simulink library "LM_LIB"  (R2019b)
settings: Solver=VariableStepAuto  StartTime=0.0  StopTime=10.0  RelTol=1e-3
undefined symbols (not defined in the file): P_LM_FusBLParFiltP, P_LM_FusParC0Index, P_LM_FusParC1Index, P_LM_FusParC2Index, P_LM_FusParC3Index, P_LM_OTLBufTPMinPntNum, P_LM_OTLBufTPSPosMinDis, P_LM_OTLRearMaxDis, P_LM_OTLTPNum
libraries: simulink x84, $bdroot x3
(part 4 of 5)

== system LM_LIB/LM_OTL_Buf2InfoUpdate/LM_OTL_BufLe1StoreInfoCalc/LM_OTL_ObjSICCurLeObj1InBufLe1 ==
  LM_OTLCurLeLaObj1RcdFlg : Inport
  LM_OTLCurLeLaObj1ID : Inport  Port=2
  LM_OTLCurLeLaObj1Dx : Inport  Port=3
  LM_OTLCurLeLaObj1Dy : Inport  Port=4
  LM_OTLBufL1PNumK1 : Inport  Port=5
  LM_OTLBufL1SPPosK1 : Inport  Port=6
  LM_OTLBufL1EPPosK1 : Inport  Port=7
  LM_OTLBufDxVectK1Adju : Inport  Port=8
  Action Port : ActionPort
  LM_OTL_BufL1DxInfo : Subsystem
  LM_OTL_BufL1DyInfo : Subsystem
  LM_OTL_BufL1EPInfo : Subsystem
  LM_OTL_BufL1IDInfo : Subsystem
  LM_OTL_BufL1PNumAndSPInfo : $bdroot/LM_OTL_Buf1InfoUpdate/LM_OTL_BufLe1StoreInfoCalc/LM_OTL_ObjSICCurLeObj1InBufLe1/LM_OTL_BufL1PNumAndSPInfo  SystemSampleTime=-1  Latency=0  AutoFrameSizeCalculation=off
  LM_OTL_BufL1UpdateFlg : Subsystem
  LM_OTLBufL1UpdateFlg : Outport
  LM_OTLBufL1ObjID : Outport  Port=2
  LM_OTLBufL1Objdx : Outport  Port=3
  LM_OTLBufL1Objdy : Outport  Port=4
  LM_OTLBufL1ObjTPNum : Outport  Port=5
  LM_OTLBufL1ObjTPSP : Outport  Port=6
  LM_OTLBufL1ObjTPEP : Outport  Port=7
  wires:
  LM_OTL_BufL1EPInfo/1(LM_OTLBufL1EPPos) -> LM_OTLBufL1ObjTPEP/1, [LM_OTLBufL1EPPos]
  [LM_OTLBufL1EPPos] -> LM_OTL_BufL1PNumAndSPInfo/4
  LM_OTL_BufL1IDInfo/1(LM_OTLBufL1ObjID) -> LM_OTLBufL1ObjID/1
  LM_OTL_BufL1DxInfo/1(LM_OTLBufL1Objdx) -> LM_OTLBufL1Objdx/1
  LM_OTL_BufL1DyInfo/1(LM_OTLBufL1ObjDy) -> LM_OTLBufL1Objdy/1
  LM_OTL_BufL1PNumAndSPInfo/1 -> LM_OTLBufL1ObjTPNum/1
  LM_OTL_BufL1PNumAndSPInfo/2 -> LM_OTLBufL1ObjTPSP/1
  LM_OTL_BufL1UpdateFlg/1(LM_OTLBufL1UpdateFlg) -> LM_OTLBufL1UpdateFlg/1
  LM_OTLCurLeLaObj1RcdFlg/1 -> LM_OTL_BufL1EPInfo/1(LM_OTLCurLeLaObj1RcdFlg), LM_OTL_BufL1PNumAndSPInfo/2, LM_OTL_BufL1DyInfo/2(LM_OTLCurLeLaObj1RcdFlg), LM_OTL_BufL1DxInfo/2(LM_OTLCurLeLaObj1RcdFlg), LM_OTL_BufL1UpdateFlg/1(LM_OTLCurLeLaObj1RcdFlg)
  LM_OTLCurLeLaObj1ID/1 -> LM_OTL_BufL1IDInfo/1(LM_OTLCurLeLaObj1ID)
  LM_OTLCurLeLaObj1Dx/1 -> LM_OTL_BufL1DxInfo/1(LM_OTLCurLeLaObj1Dx)
  LM_OTLCurLeLaObj1Dy/1 -> LM_OTL_BufL1DyInfo/1(LM_OTLCurLeLaObj1Dy)
  LM_OTLBufL1PNumK1/1 -> LM_OTL_BufL1PNumAndSPInfo/1
  LM_OTLBufL1SPPosK1/1 -> LM_OTL_BufL1PNumAndSPInfo/3
  LM_OTLBufL1EPPosK1/1 -> LM_OTL_BufL1EPInfo/2(LM_OTLBufL1EPPosK1)
  LM_OTLBufDxVectK1Adju/1 -> LM_OTL_BufL1PNumAndSPInfo/5

== system LM_LIB/LM_OTL_Buf2InfoUpdate/LM_OTL_BufLe1StoreInfoCalc/LM_OTL_ObjSICCurLeObj2InBufLe1 ==
  LM_OTLCurLeLaObj2RcdFlg : Inport
  LM_OTLCurLeLaObj2ID : Inport  Port=2
  LM_OTLCurLeLaObj2Dx : Inport  Port=3
  LM_OTLCurLeLaObj2Dy : Inport  Port=4
  LM_OTLBufL1PNumK1 : Inport  Port=5
  LM_OTLBufL1SPPosK1 : Inport  Port=6
  LM_OTLBufL1EPPosK1 : Inport  Port=7
  LM_OTLBufDxVectK1Adju : Inport  Port=8
  Action Port : ActionPort
  LM_OTL_BufL1DxInfo : Subsystem
  LM_OTL_BufL1DyInfo : Subsystem
  LM_OTL_BufL1EPInfo : Subsystem
  LM_OTL_BufL1IDInfo : Subsystem
  LM_OTL_BufL1PNumAndSPInfo : $bdroot/LM_OTL_Buf1InfoUpdate/LM_OTL_BufLe1StoreInfoCalc/LM_OTL_ObjSICCurLeObj1InBufLe1/LM_OTL_BufL1PNumAndSPInfo  SystemSampleTime=-1  Latency=0  AutoFrameSizeCalculation=off
  LM_OTL_BufL1UpdateFlg : Subsystem
  LM_OTLBufL1UpdateFlg : Outport
  LM_OTLBufL1ObjID : Outport  Port=2
  LM_OTLBufL1Objdx : Outport  Port=3
  LM_OTLBufL1Objdy : Outport  Port=4
  LM_OTLBufL1ObjTPNum : Outport  Port=5
  LM_OTLBufL1ObjTPSP : Outport  Port=6
  LM_OTLBufL1ObjTPEP : Outport  Port=7
  wires:
  LM_OTLBufL1PNumK1/1 -> LM_OTL_BufL1PNumAndSPInfo/1
  LM_OTLCurLeLaObj2Dx/1 -> LM_OTL_BufL1DxInfo/1(LM_OTLCurLeLaObj1Dx)
  LM_OTL_BufL1IDInfo/1(LM_OTLBufL1ObjID) -> LM_OTLBufL1ObjID/1
  [LM_OTLBufL1EPPos] -> LM_OTL_BufL1PNumAndSPInfo/4
  LM_OTL_BufL1PNumAndSPInfo/1 -> LM_OTLBufL1ObjTPNum/1
  LM_OTLCurLeLaObj2Dy/1 -> LM_OTL_BufL1DyInfo/1(LM_OTLCurLeLaObj1Dy)
  LM_OTL_BufL1DxInfo/1(LM_OTLBufL1Objdx) -> LM_OTLBufL1Objdx/1
  LM_OTLCurLeLaObj2RcdFlg/1 -> LM_OTL_BufL1EPInfo/1(LM_OTLCurLeLaObj1RcdFlg), LM_OTL_BufL1PNumAndSPInfo/2, LM_OTL_BufL1DyInfo/2(LM_OTLCurLeLaObj1RcdFlg), LM_OTL_BufL1DxInfo/2(LM_OTLCurLeLaObj1RcdFlg), LM_OTL_BufL1UpdateFlg/1(LM_OTLCurLeLaObj1RcdFlg)
  LM_OTL_BufL1PNumAndSPInfo/2 -> LM_OTLBufL1ObjTPSP/1
  LM_OTLCurLeLaObj2ID/1 -> LM_OTL_BufL1IDInfo/1(LM_OTLCurLeLaObj1ID)
  LM_OTL_BufL1DyInfo/1(LM_OTLBufL1ObjDy) -> LM_OTLBufL1Objdy/1
  LM_OTL_BufL1EPInfo/1(LM_OTLBufL1EPPos) -> LM_OTLBufL1ObjTPEP/1, [LM_OTLBufL1EPPos]
  LM_OTLBufL1EPPosK1/1 -> LM_OTL_BufL1EPInfo/2(LM_OTLBufL1EPPosK1)
  LM_OTL_BufL1UpdateFlg/1(LM_OTLBufL1UpdateFlg) -> LM_OTLBufL1UpdateFlg/1
  LM_OTLBufL1SPPosK1/1 -> LM_OTL_BufL1PNumAndSPInfo/3
  LM_OTLBufDxVectK1Adju/1 -> LM_OTL_BufL1PNumAndSPInfo/5

== system LM_LIB/LM_OTL_Buf2InfoUpdate/LM_OTL_BufLe1StoreInfoCalc/LM_OTL_ObjSICNoCurObjInBufLe1 ==
  LM_OTLCurLeLaObj1Index : Inport
  LM_OTLCurLeLaObj2Index : Inport  Port=2
  LM_OTLCurLeLaObj1RcdedFlg : Inport  Port=3
  LM_OTLCurLeLaObj1ID : Inport  Port=4
  LM_OTLCurLeLaObj2ID : Inport  Port=5
  LM_OTLCurLeLaObj1Dx : Inport  Port=6
  LM_OTLCurLeLaObj2Dx : Inport  Port=7
  LM_OTLCurLeLaObj1Dy : Inport  Port=8
  LM_OTLCurLeLaObj2Dy : Inport  Port=9
  LM_OTLBufL1LastTPValid : Inport  Port=10
  LM_OTLBufL1LastEPPos : Inport  Port=11
  LM_OTLBuf1ID : Inport  Port=12
  Action Port : ActionPort
  LM_OTL_BufL1IDInfo : Subsystem
  LM_OTL_BufL1PNumInfo : Subsystem
  LM_OTL_BufL1SPInfo : Subsystem
  LM_OTL_BufL2EPInfo : Subsystem
  LM_OTL_BufL2PosInfo : Subsystem
  LM_OTLBufL2UpdateFlg : Outport
  LM_OTLBufL2ObjID : Outport  Port=2
  LM_OTLBufL2Objdx : Outport  Port=3
  LM_OTLBufL2Objdy : Outport  Port=4
  LM_OTLBufL2ObjTPNum : Outport  Port=5
  LM_OTLBufL2ObjTPSP : Outport  Port=6
  LM_OTLBufL2ObjTPEP : Outport  Port=7
  wires:
  LM_OTL_BufL1IDInfo/2(LM_OTLBufL2ObjID) -> LM_OTLBufL2ObjID/1, LM_OTL_BufL2PosInfo/1(LM_OTLBufL2ObjID), LM_OTL_BufL1PNumInfo/1(LM_OTLBufL2ObjID), LM_OTL_BufL1SPInfo/1(LM_OTLBufL2ObjID)
  LM_OTL_BufL2PosInfo/1(LM_OTLBufL2Objdx) -> LM_OTLBufL2Objdx/1
  LM_OTL_BufL1PNumInfo/1(LM_OTLBufL1TPNum) -> LM_OTLBufL2ObjTPNum/1
  LM_OTL_BufL1SPInfo/1(LM_OTLBufL2SPPos) -> LM_OTL_BufL2EPInfo/1(LM_OTLBufL2SPPos), LM_OTLBufL2ObjTPSP/1
  LM_OTL_BufL2EPInfo/1(LM_OTLBufL2EPPos) -> LM_OTLBufL2ObjTPEP/1
  LM_OTLCurLeLaObj1Index/1 -> LM_OTL_BufL1IDInfo/2(LM_OTLCurLeLaObj1Index)
  LM_OTLCurLeLaObj2Index/1 -> LM_OTL_BufL1IDInfo/3(LM_OTLCurLeLaObj2Index)
  LM_OTLCurLeLaObj1RcdedFlg/1 -> LM_OTL_BufL1IDInfo/4(LM_OTLCurLeLaObj1RcdedFlg)
  LM_OTLCurLeLaObj1ID/1 -> LM_OTL_BufL2PosInfo/2(LM_OTLCurLeLaObj1ID), LM_OTL_BufL1IDInfo/5(LM_OTLCurLeLaObj1ID)
  LM_OTLCurLeLaObj2ID/1 -> LM_OTL_BufL2PosInfo/3(LM_OTLCurLeLaObj2ID), LM_OTL_BufL1IDInfo/6(LM_OTLCurLeLaObj2ID)
  LM_OTLCurLeLaObj1Dx/1 -> LM_OTL_BufL2PosInfo/4(LM_OTLCurLeLaObj1Dx)
  LM_OTLCurLeLaObj2Dx/1 -> LM_OTL_BufL2PosInfo/5(LM_OTLCurLeLaObj2Dx)
  LM_OTLBufL1LastTPValid/1 -> LM_OTL_BufL1SPInfo/2(LM_OTLBufL2LastTPValid)
  LM_OTLBufL1LastEPPos/1 -> LM_OTL_BufL1SPInfo/3(LM_OTLBufL2LastEPPos)
  LM_OTL_BufL1IDInfo/1(LM_OTLBufL2UpdateFlg) -> LM_OTLBufL2UpdateFlg/1
  LM_OTLBuf1ID/1 -> LM_OTL_BufL1IDInfo/1(LM_OTLBuf1ID)
  LM_OTL_BufL2PosInfo/2(LM_OTLBufL2Objdy) -> LM_OTLBufL2Objdy/1
  LM_OTLCurLeLaObj1Dy/1 -> LM_OTL_BufL2PosInfo/6(LM_OTLCurLeLaObj1Dy)
  LM_OTLCurLeLaObj2Dy/1 -> LM_OTL_BufL2PosInfo/7(LM_OTLCurLeLaObj2Dy)

== system LM_LIB/LM_OTLBuf1InfoNew/LM_OTL_BufLe1StoreInfoCalc/LM_OTL_ObjSICCurLeObj1InBufLe1/LM_OTL_BufL1DxInfo ==
  LM_OTLCurLeLaObj1Dx : Inport
  LM_OTLCurLeLaObj1RcdFlg : Inport  Port=2
  Constant : Constant  Value=0  OutDataTypeStr=single
  Switch4 : Switch  Criteria=u2 ~= 0
  LM_OTLBufL1Objdx : Outport
  wires:
  LM_OTLCurLeLaObj1Dx/1 -> Switch4/1
  LM_OTLCurLeLaObj1RcdFlg/1 -> Switch4/2
  Switch4/1 -> LM_OTLBufL1Objdx/1  "LM_OTLBufL1Objdx"
  Constant/1 -> Switch4/3

== system LM_LIB/LM_OTLBuf1InfoNew/LM_OTL_BufLe1StoreInfoCalc/LM_OTL_ObjSICCurLeObj1InBufLe1/LM_OTL_BufL1DyInfo ==
  LM_OTLCurLeLaObj1Dy : Inport
  LM_OTLCurLeLaObj1RcdFlg : Inport  Port=2
  LM_OTLCurLeLaObj1Dx : Inport  Port=3
  LM_OTLCurEgoLaObj1DyVar : Inport  Port=4
  LM_OTLCurEgoLaObj1Vy : Inport  Port=5
  LM_OTLCurEgoLaObj1VyVar : Inport  Port=6
  LM_OTLBufEgo1DyFiltHistK : Inport  Port=7
  LM_OTLBufEgo1DyVarHistK : Inport  Port=8
  psiDt : Inport  Port=9
  tDt : Inport  Port=10
  Constant : Constant  Value=0  OutDataTypeStr=single
  MATLAB Function : MATLAB Function  TreatAsAtomicUnit=on
  Switch1 : Switch  Criteria=u2 ~= 0
  Switch4 : Switch  Criteria=u2 ~= 0
  LM_OTLBufL1ObjDy : Outport
  LM_OTLBufEgo1DyVarHist : Outport  Port=2
  wires:
  Constant/1 -> Switch4/3
  Switch4/1 -> LM_OTLBufL1ObjDy/1  "LM_OTLBufL1ObjDy"
  LM_OTLCurLeLaObj1Dy/1 -> MATLAB Function/2(dy)
  LM_OTLCurLeLaObj1RcdFlg/1 -> Switch1/2, Switch4/2
  LM_OTLCurEgoLaObj1DyVar/1 -> MATLAB Function/3(varDy)
  LM_OTLCurEgoLaObj1Vy/1 -> MATLAB Function/4(vy)
  LM_OTLCurEgoLaObj1VyVar/1 -> MATLAB Function/5(varVy)
  LM_OTLCurLeLaObj1Dx/1 -> MATLAB Function/1(dx)
  LM_OTLBufEgo1DyFiltHistK/1 -> MATLAB Function/8(dyHist)
  LM_OTLBufEgo1DyVarHistK/1 -> Switch1/3, MATLAB Function/9(varDyHist)
  Switch1/1 -> LM_OTLBufEgo1DyVarHist/1  "LM_OTLBufL1ObjDy"
  MATLAB Function/2(varDyFilt) -> Switch1/1
  MATLAB Function/1(dyFilt) -> Switch4/1
  psiDt/1 -> MATLAB Function/6(psiDt)
  tDt/1 -> MATLAB Function/7(tDt)

== system LM_LIB/LM_OTLBuf1InfoNew/LM_OTL_BufLe1StoreInfoCalc/LM_OTL_ObjSICCurLeObj1InBufLe1/LM_OTL_BufL1EPInfo ==
  note: P_LM_OTLTPNum
  LM_OTLCurLeLaObj1RcdFlg : Inport
  LM_OTLBufL1EPPosK1 : Inport  Port=2
  Add : Sum
  Constant : Constant  OutDataTypeStr=uint8
  Constant1 : Constant  Value=P_LM_OTLTPNum  OutDataTypeStr=uint8
  Constant2 : Constant  OutDataTypeStr=uint8
  Relational Operator : RelationalOperator  Operator=>  OutDataTypeStr=boolean  RndMeth=Simplest
  Switch1 : Switch  Criteria=u2 ~= 0
  Switch4 : Switch  Criteria=u2 ~= 0
  LM_OTLBufL1EPPos : Outport
  wires:
  Constant/1 -> Add/2
  LM_OTLCurLeLaObj1RcdFlg/1 -> Switch4/2
  LM_OTLBufL1EPPosK1/1 -> Switch4/3, Add/1
  Switch1/1 -> LM_OTLBufL1EPPos/1  "LM_OTLBufL1EPPos"
  Relational Operator/1 -> Switch1/2
  Switch4/1 -> Switch1/3, Relational Operator/1
  Constant1/1 -> Relational Operator/2
  Constant2/1 -> Switch1/1
  Add/1 -> Switch4/1

== system LM_LIB/LM_OTLBuf1InfoNew/LM_OTL_BufLe1StoreInfoCalc/LM_OTL_ObjSICCurLeObj1InBufLe1/LM_OTL_BufL1IDInfo ==
  LM_OTLCurLeLaObj1ID : Inport
  Signal Conversion : SignalConversion  OverrideOpt=off
  LM_OTLBufL1ObjID : Outport
  wires:
  LM_OTLCurLeLaObj1ID/1 -> Signal Conversion/1
  Signal Conversion/1 -> LM_OTLBufL1ObjID/1  "LM_OTLBufL1ObjID"

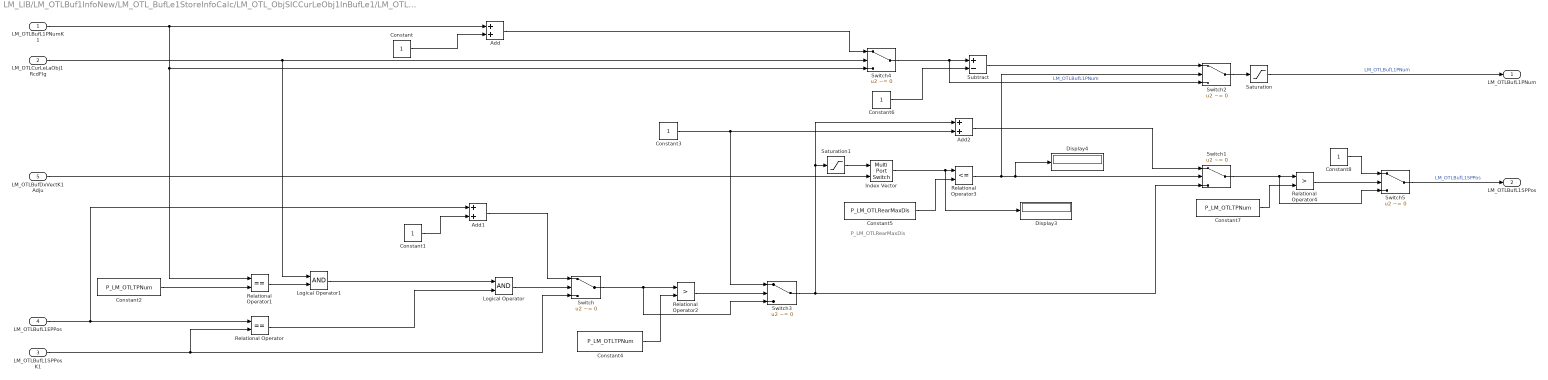
== system LM_LIB/LM_OTLBuf1InfoNew/LM_OTL_BufLe1StoreInfoCalc/LM_OTL_ObjSICCurLeObj1InBufLe1/LM_OTL_BufL1PNumAndSPInfo ==
  note: P_LM_OTLRearMaxDis
  LM_OTLBufL1PNumK1 : Inport
  LM_OTLCurLeLaObj1RcdFlg : Inport  Port=2
  LM_OTLBufL1SPPosK1 : Inport  Port=3
  LM_OTLBufL1EPPos : Inport  Port=4
  LM_OTLBufDxVectK1Adju : Inport  Port=5
  Add : Sum
  Add1 : Sum
  Add2 : Sum
  Constant{,1,3,6,8} (5 alike) : Constant  OutDataTypeStr=uint8
  Constant2 : Constant  Value=P_LM_OTLTPNum  OutDataTypeStr=uint8
  Constant4 : Constant  Value=P_LM_OTLTPNum  OutDataTypeStr=uint8
  Constant5 : Constant  Value=P_LM_OTLRearMaxDis
  Constant7 : Constant  Value=P_LM_OTLTPNum  OutDataTypeStr=uint8
  Display3 : Display
  Display4 : Display
  Index Vector : MultiPortSwitch  Inputs=1
  Logical Operator : Logic  AllPortsSameDT=off  OutDataTypeStr=boolean
  Logical Operator1 : Logic  AllPortsSameDT=off  OutDataTypeStr=boolean
  Relational Operator : RelationalOperator  Operator===  OutDataTypeStr=boolean  RndMeth=Simplest
  Relational Operator1 : RelationalOperator  Operator===  OutDataTypeStr=boolean  RndMeth=Simplest
  Relational Operator2 : RelationalOperator  Operator=>  OutDataTypeStr=boolean  RndMeth=Simplest
  Relational Operator3 : RelationalOperator  Operator=<=  OutDataTypeStr=boolean  RndMeth=Simplest
  Relational Operator4 : RelationalOperator  Operator=>  OutDataTypeStr=boolean  RndMeth=Simplest
  Saturation : Saturate  UpperLimit=80  LowerLimit=0
  Saturation1 : Saturate  UpperLimit=80  LowerLimit=0
  Subtract : Sum  Inputs=+-
  Switch{,1..5} (6 alike) : Switch  Criteria=u2 ~= 0
  LM_OTLBufL1PNum : Outport
  LM_OTLBufL1SPPos : Outport  Port=2
  wires:
  Saturation/1 -> LM_OTLBufL1PNum/1  "LM_OTLBufL1PNum"
  LM_OTLCurLeLaObj1RcdFlg/1 -> Logical Operator1/1, Switch4/2
  Switch2/1 -> Saturation/1
  Constant/1 -> Add/2
  Add/1 -> Switch4/1
  Constant2/1 -> Relational Operator1/2
  Constant3/1 -> Switch3/1, Add2/2
  Constant4/1 -> Relational Operator2/2
  Add1/1 -> Switch/1
  Switch/1 -> Switch3/3, Relational Operator2/1
  Relational Operator2/1 -> Switch3/2
  LM_OTLBufL1SPPosK1/1 -> Switch/3, Relational Operator/2
  Relational Operator1/1 -> Logical Operator1/2
  Logical Operator/1 -> Switch/2
  LM_OTLBufL1EPPos/1 -> Relational Operator/1, Add1/1
  Relational Operator/1 -> Logical Operator/2
  LM_OTLBufL1PNumK1/1 -> Add/1, Relational Operator1/1, Switch4/3
  Switch3/1 -> Switch1/3, Add2/1, Saturation1/1
  Constant1/1 -> Add1/2
  LM_OTLBufDxVectK1Adju/1 -> Index Vector/2
  Index Vector/1 -> Display3/1, Relational Operator3/1
  Constant5/1 -> Relational Operator3/2
  Relational Operator3/1 -> Switch2/2, Display4/1, Switch1/2
  Switch5/1 -> LM_OTLBufL1SPPos/1  "LM_OTLBufL1SPPos"
  Add2/1 -> Switch1/1
  Subtract/1 -> Switch2/1
  Saturation1/1 -> Index Vector/1
  Logical Operator1/1 -> Logical Operator/1
  Switch4/1 -> Switch2/3, Subtract/1  "LM_OTLBufL1PNum"
  Constant6/1 -> Subtract/2
  Switch1/1 -> Switch5/3, Relational Operator4/1
  Relational Operator4/1 -> Switch5/2
  Constant7/1 -> Relational Operator4/2
  Constant8/1 -> Switch5/1

== system LM_LIB/LM_OTLBuf1InfoNew/LM_OTL_BufLe1StoreInfoCalc/LM_OTL_ObjSICCurLeObj1InBufLe1/LM_OTL_BufL1UpdateFlg ==
  LM_OTLCurLeLaObj1RcdFlg : Inport
  Signal Conversion : SignalConversion  OverrideOpt=off
  LM_OTLBufL1UpdateFlg : Outport
  wires:
  LM_OTLCurLeLaObj1RcdFlg/1 -> Signal Conversion/1
  Signal Conversion/1 -> LM_OTLBufL1UpdateFlg/1  "LM_OTLBufL1UpdateFlg"

== system LM_LIB/LM_OTLBuf1InfoNew/LM_OTL_BufLe1StoreInfoCalc/LM_OTL_ObjSICCurLeObj2InBufLe1/LM_OTL_BufL1DxInfo ==
  LM_OTLCurLeLaObj1Dx : Inport
  LM_OTLCurLeLaObj1RcdFlg : Inport  Port=2
  Constant : Constant  Value=0  OutDataTypeStr=single
  Switch4 : Switch  Criteria=u2 ~= 0
  LM_OTLBufL1Objdx : Outport
  wires:
  LM_OTLCurLeLaObj1Dx/1 -> Switch4/1
  LM_OTLCurLeLaObj1RcdFlg/1 -> Switch4/2
  Switch4/1 -> LM_OTLBufL1Objdx/1  "LM_OTLBufL1Objdx"
  Constant/1 -> Switch4/3

== system LM_LIB/LM_OTLBuf1InfoNew/LM_OTL_BufLe1StoreInfoCalc/LM_OTL_ObjSICCurLeObj2InBufLe1/LM_OTL_BufL1DyInfo ==
  LM_OTLCurEgoLaObj2Dx : Inport
  LM_OTLCurLeLaObj1Dy : Inport  Port=2
  LM_OTLCurLeLaObj1RcdFlg : Inport  Port=3
  LM_OTLCurEgoLaObj2DyVar : Inport  Port=4
  LM_OTLCurEgoLaObj2Vy : Inport  Port=5
  LM_OTLCurEgoLaObj2VyVar : Inport  Port=6
  LM_OTLBufEgo1DyFiltHistK : Inport  Port=7
  LM_OTLBufEgo1DyVarHistK : Inport  Port=8
  psiDt : Inport  Port=9
  tDt : Inport  Port=10
  Constant : Constant  Value=0  OutDataTypeStr=single
  MATLAB Function : MATLAB Function  TreatAsAtomicUnit=on
  Switch1 : Switch  Criteria=u2 ~= 0
  Switch4 : Switch  Criteria=u2 ~= 0
  LM_OTLBufL1ObjDy : Outport
  LM_OTLBufEgo1DyVarHist : Outport  Port=2
  wires:
  Constant/1 -> Switch4/3
  Switch4/1 -> LM_OTLBufL1ObjDy/1  "LM_OTLBufL1ObjDy"
  LM_OTLCurLeLaObj1Dy/1 -> MATLAB Function/2(dy)
  LM_OTLCurLeLaObj1RcdFlg/1 -> Switch1/2, Switch4/2
  LM_OTLCurEgoLaObj2VyVar/1 -> MATLAB Function/5(varVy)
  LM_OTLCurEgoLaObj2Vy/1 -> MATLAB Function/4(vy)
  LM_OTLCurEgoLaObj2DyVar/1 -> MATLAB Function/3(varDy)
  LM_OTLCurEgoLaObj2Dx/1 -> MATLAB Function/1(dx)
  MATLAB Function/1(dyFilt) -> Switch4/1
  MATLAB Function/2(varDyFilt) -> Switch1/1
  LM_OTLBufEgo1DyVarHistK/1 -> Switch1/3, MATLAB Function/9(varDyHist)
  psiDt/1 -> MATLAB Function/6(psiDt)
  tDt/1 -> MATLAB Function/7(tDt)
  LM_OTLBufEgo1DyFiltHistK/1 -> MATLAB Function/8(dyHist)
  Switch1/1 -> LM_OTLBufEgo1DyVarHist/1  "LM_OTLBufEgo1DyVarHist"

== system LM_LIB/LM_OTLBuf1InfoNew/LM_OTL_BufLe1StoreInfoCalc/LM_OTL_ObjSICCurLeObj2InBufLe1/LM_OTL_BufL1EPInfo ==
  note: P_LM_OTLTPNum
  LM_OTLCurLeLaObj1RcdFlg : Inport
  LM_OTLBufL1EPPosK1 : Inport  Port=2
  Add : Sum
  Constant : Constant  OutDataTypeStr=uint8
  Constant1 : Constant  Value=80  OutDataTypeStr=uint8
  Constant2 : Constant  OutDataTypeStr=uint8
  Relational Operator : RelationalOperator  Operator=>  OutDataTypeStr=boolean  RndMeth=Simplest
  Switch1 : Switch  Criteria=u2 ~= 0
  Switch4 : Switch  Criteria=u2 ~= 0
  LM_OTLBufL1EPPos : Outport
  wires:
  Constant/1 -> Add/2
  LM_OTLCurLeLaObj1RcdFlg/1 -> Switch4/2
  LM_OTLBufL1EPPosK1/1 -> Switch4/3, Add/1
  Switch1/1 -> LM_OTLBufL1EPPos/1  "LM_OTLBufL1EPPos"
  Relational Operator/1 -> Switch1/2
  Switch4/1 -> Switch1/3, Relational Operator/1
  Constant1/1 -> Relational Operator/2
  Constant2/1 -> Switch1/1
  Add/1 -> Switch4/1

== system LM_LIB/LM_OTLBuf1InfoNew/LM_OTL_BufLe1StoreInfoCalc/LM_OTL_ObjSICCurLeObj2InBufLe1/LM_OTL_BufL1IDInfo ==
  LM_OTLCurLeLaObj1ID : Inport
  Signal Conversion : SignalConversion  OverrideOpt=off
  LM_OTLBufL1ObjID : Outport
  wires:
  LM_OTLCurLeLaObj1ID/1 -> Signal Conversion/1
  Signal Conversion/1 -> LM_OTLBufL1ObjID/1  "LM_OTLBufL1ObjID"

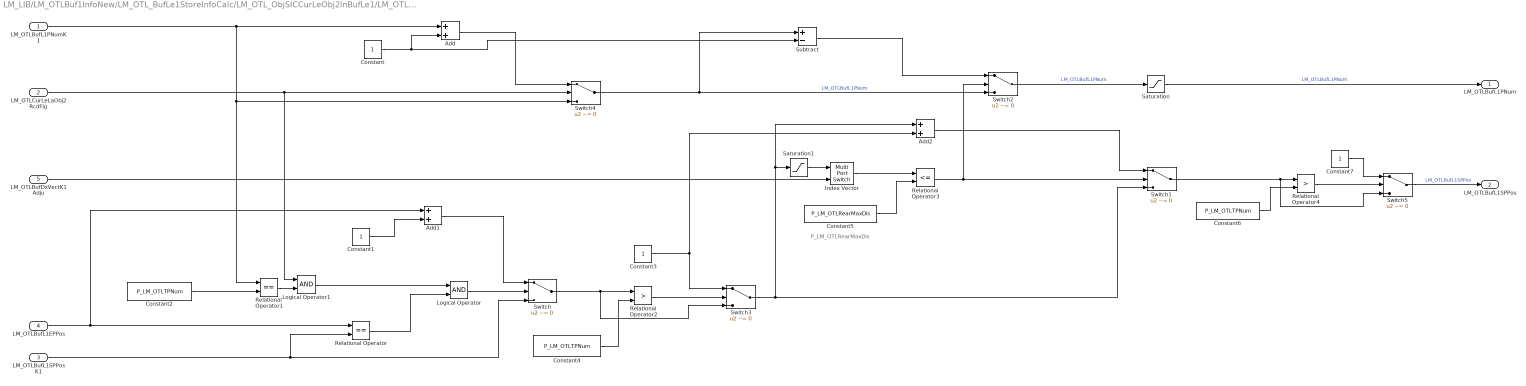
== system LM_LIB/LM_OTLBuf1InfoNew/LM_OTL_BufLe1StoreInfoCalc/LM_OTL_ObjSICCurLeObj2InBufLe1/LM_OTL_BufL1PNumAndSPInfo ==
  note: P_LM_OTLRearMaxDis
  LM_OTLBufL1PNumK1 : Inport
  LM_OTLCurLeLaObj2RcdFlg : Inport  Port=2
  LM_OTLBufL1SPPosK1 : Inport  Port=3
  LM_OTLBufL1EPPos : Inport  Port=4
  LM_OTLBufDxVectK1Adju : Inport  Port=5
  Add : Sum
  Add1 : Sum
  Add2 : Sum
  Constant{,1,3,7} (4 alike) : Constant  OutDataTypeStr=uint8
  Constant2 : Constant  Value=P_LM_OTLTPNum  OutDataTypeStr=uint8
  Constant4 : Constant  Value=P_LM_OTLTPNum  OutDataTypeStr=uint8
  Constant5 : Constant  Value=P_LM_OTLRearMaxDis
  Constant6 : Constant  Value=P_LM_OTLTPNum  OutDataTypeStr=uint8
  Index Vector : MultiPortSwitch  Inputs=1
  Logical Operator : Logic  AllPortsSameDT=off  OutDataTypeStr=boolean
  Logical Operator1 : Logic  AllPortsSameDT=off  OutDataTypeStr=boolean
  Relational Operator : RelationalOperator  Operator===  OutDataTypeStr=boolean  RndMeth=Simplest
  Relational Operator1 : RelationalOperator  Operator===  OutDataTypeStr=boolean  RndMeth=Simplest
  Relational Operator2 : RelationalOperator  Operator=>  OutDataTypeStr=boolean  RndMeth=Simplest
  Relational Operator3 : RelationalOperator  Operator=<=  OutDataTypeStr=boolean  RndMeth=Simplest
  Relational Operator4 : RelationalOperator  Operator=>  OutDataTypeStr=boolean  RndMeth=Simplest
  Saturation : Saturate  UpperLimit=80  LowerLimit=0
  Saturation1 : Saturate  UpperLimit=80  LowerLimit=1
  Subtract : Sum  Inputs=+-
  Switch{,1..5} (6 alike) : Switch  Criteria=u2 ~= 0
  LM_OTLBufL1PNum : Outport
  LM_OTLBufL1SPPos : Outport  Port=2
  wires:
  Switch5/1 -> LM_OTLBufL1SPPos/1  "LM_OTLBufL1SPPos"
  LM_OTLBufL1PNumK1/1 -> Add/1, Switch4/3, Relational Operator1/1
  LM_OTLBufL1SPPosK1/1 -> Switch/3, Relational Operator/2
  Relational Operator2/1 -> Switch3/2
  Switch/1 -> Switch3/3, Relational Operator2/1
  Constant3/1 -> Add2/2, Switch3/1
  Relational Operator/1 -> Logical Operator/2
  Add1/1 -> Switch/1
  Relational Operator1/1 -> Logical Operator1/2
  Relational Operator3/1 -> Switch2/2, Switch1/2
  Add2/1 -> Switch1/1
  Index Vector/1 -> Relational Operator3/1
  LM_OTLBufL1EPPos/1 -> Relational Operator/1, Add1/1
  Constant1/1 -> Add1/2
  Constant/1 -> Subtract/2, Add/2
  LM_OTLCurLeLaObj2RcdFlg/1 -> Logical Operator1/1, Switch4/2
  Saturation/1 -> LM_OTLBufL1PNum/1  "LM_OTLBufL1PNum"
  Constant4/1 -> Relational Operator2/2
  Constant5/1 -> Relational Operator3/2
  Switch3/1 -> Switch1/3, Add2/1, Saturation1/1
  LM_OTLBufDxVectK1Adju/1 -> Index Vector/2
  Logical Operator/1 -> Switch/2
  Subtract/1 -> Switch2/1
  Saturation1/1 -> Index Vector/1
  Constant2/1 -> Relational Operator1/2
  Logical Operator1/1 -> Logical Operator/1
  Add/1 -> Switch4/1
  Switch2/1 -> Saturation/1  "LM_OTLBufL1PNum"
  Switch4/1 -> Subtract/1, Switch2/3  "LM_OTLBufL1PNum"
  Switch1/1 -> Switch5/3, Relational Operator4/1
  Relational Operator4/1 -> Switch5/2
  Constant6/1 -> Relational Operator4/2
  Constant7/1 -> Switch5/1

== system LM_LIB/LM_OTLBuf1InfoNew/LM_OTL_BufLe1StoreInfoCalc/LM_OTL_ObjSICCurLeObj2InBufLe1/LM_OTL_BufL1UpdateFlg ==
  LM_OTLCurLeLaObj1RcdFlg : Inport
  Signal Conversion : SignalConversion  OverrideOpt=off
  LM_OTLBufL1UpdateFlg : Outport
  wires:
  LM_OTLCurLeLaObj1RcdFlg/1 -> Signal Conversion/1
  Signal Conversion/1 -> LM_OTLBufL1UpdateFlg/1  "LM_OTLBufL1UpdateFlg"

== system LM_LIB/LM_OTLBuf1InfoNew/LM_OTL_BufLe1StoreInfoCalc/LM_OTL_ObjSICNoCurObjInBufLe1/LM_OTL_BufL1DxInfo ==
  LM_OTLCurLeLaObj1Index : Inport
  LM_OTLCurLeLaObj2Index : Inport  Port=2
  LM_OTLCurLeLaObj1RcdedFlg : Inport  Port=3
  LM_OTLCurLeLaObj1Dx : Inport  Port=4
  LM_OTLCurLeLaObj2Dx : Inport  Port=5
  Compare To Zero : simulink/Logic and Bit Operations/Compare To Zero  relop===  OutDataTypeStr=boolean
  Compare To Zero1 : simulink/Logic and Bit Operations/Compare To Zero  relop===  OutDataTypeStr=boolean
  Compare To Zero2 : simulink/Logic and Bit Operations/Compare To Zero  relop===  OutDataTypeStr=boolean
  Constant : Constant  Value=0  OutDataTypeStr=single
  Constant1 : Constant  Value=0  OutDataTypeStr=single
  DocBlock : simulink/Model-Wide Utilities/DocBlock  DocumentType=Text
      content=|
      | 1. 功能描述
      |    该模块主要功能
      | 2. 算法说明
      | 2.1 当左车道最近目标索引为0时，即左车道无目标，输出0
      | 2.2 当左车道最近目标索引不为0时
      |     2.2.1 如果左车道最近目标ID未在buffer中存储，则输出左车道最近目标的dx
      |     2.2.2 如果左车道最近目标ID已经在buffer中存储
      |           2.2.2.1 如果左车道第二近目标ID不为0，则输出左车道第二近目标dx
      |           2.2.2.2 如果左车道第二近目标ID为0，则输出0
  Switch1 : Switch  Criteria=u2 ~= 0
  Switch2 : Switch  Criteria=u2 ~= 0
  Switch4 : Switch  Criteria=u2 ~= 0
  LM_OTLBufL1Objdx : Outport
  wires:
  LM_OTLCurLeLaObj1RcdedFlg/1 -> Compare To Zero1/1
  Switch1/1 -> Switch4/3
  Switch4/1 -> LM_OTLBufL1Objdx/1  "LM_OTLBufL1Objdx"
  LM_OTLCurLeLaObj1Index/1 -> Compare To Zero/1
  LM_OTLCurLeLaObj2Index/1 -> Compare To Zero2/1
  Compare To Zero/1 -> Switch4/2
  Constant/1 -> Switch4/1
  Compare To Zero1/1 -> Switch1/2
  LM_OTLCurLeLaObj1Dx/1 -> Switch1/1
  Compare To Zero2/1 -> Switch2/2
  Constant1/1 -> Switch2/1
  Switch2/1 -> Switch1/3
  LM_OTLCurLeLaObj2Dx/1 -> Switch2/3

== system LM_LIB/LM_OTLBuf1InfoNew/LM_OTL_BufLe1StoreInfoCalc/LM_OTL_ObjSICNoCurObjInBufLe1/LM_OTL_BufL1DyInfo ==
  LM_OTLCurLeLaObj1Index : Inport
  LM_OTLCurLeLaObj2Index : Inport  Port=2
  LM_OTLCurLeLaObj1RcdedFlg : Inport  Port=3
  LM_OTLCurLeLaObj1Dy : Inport  Port=4
  LM_OTLCurLeLaObj2Dy : Inport  Port=5
  Compare To Zero : simulink/Logic and Bit Operations/Compare To Zero  relop===  OutDataTypeStr=boolean
  Compare To Zero1 : simulink/Logic and Bit Operations/Compare To Zero  relop===  OutDataTypeStr=boolean
  Compare To Zero2 : simulink/Logic and Bit Operations/Compare To Zero  relop===  OutDataTypeStr=boolean
  Constant : Constant  Value=0  OutDataTypeStr=single
  Constant1 : Constant  Value=0  OutDataTypeStr=single
  Switch1 : Switch  Criteria=u2 ~= 0
  Switch2 : Switch  Criteria=u2 ~= 0
  Switch4 : Switch  Criteria=u2 ~= 0
  LM_OTLBufL1Objdy : Outport
  wires:
  Constant/1 -> Switch4/1
  LM_OTLCurLeLaObj1Dy/1 -> Switch1/1
  Compare To Zero1/1 -> Switch1/2
  LM_OTLCurLeLaObj1Index/1 -> Compare To Zero/1
  Switch1/1 -> Switch4/3
  Switch4/1 -> LM_OTLBufL1Objdy/1  "LM_OTLBufL1Objdy"
  Compare To Zero/1 -> Switch4/2
  Constant1/1 -> Switch2/1
  LM_OTLCurLeLaObj1RcdedFlg/1 -> Compare To Zero1/1
  LM_OTLCurLeLaObj2Index/1 -> Compare To Zero2/1
  LM_OTLCurLeLaObj2Dy/1 -> Switch2/3
  Compare To Zero2/1 -> Switch2/2
  Switch2/1 -> Switch1/3

== system LM_LIB/LM_OTLBuf1InfoNew/LM_OTL_BufLe1StoreInfoCalc/LM_OTL_ObjSICNoCurObjInBufLe1/LM_OTL_BufL1DyInfo1 ==
  LM_OTLCurLeLaObj1Index : Inport
  LM_OTLCurLeLaObj2Index : Inport  Port=2
  LM_OTLCurLeLaObj1RcdedFlg : Inport  Port=3
  LM_OTLCurEgoLaObj1DyVar : Inport  Port=4
  LM_OTLCurEgoLaObj2DyVar : Inport  Port=5
  Compare To Zero : simulink/Logic and Bit Operations/Compare To Zero  relop===  OutDataTypeStr=boolean
  Compare To Zero1 : simulink/Logic and Bit Operations/Compare To Zero  relop===  OutDataTypeStr=boolean
  Compare To Zero2 : simulink/Logic and Bit Operations/Compare To Zero  relop===  OutDataTypeStr=boolean
  Constant : Constant  Value=0  OutDataTypeStr=single
  Constant1 : Constant  Value=0  OutDataTypeStr=single
  Switch1 : Switch  Criteria=u2 ~= 0
  Switch2 : Switch  Criteria=u2 ~= 0
  Switch4 : Switch  Criteria=u2 ~= 0
  LM_OTLBufEgo1DyVarHist : Outport
  wires:
  Switch2/1 -> Switch1/3
  Compare To Zero2/1 -> Switch2/2
  LM_OTLCurEgoLaObj2DyVar/1 -> Switch2/3
  LM_OTLCurLeLaObj2Index/1 -> Compare To Zero2/1
  LM_OTLCurLeLaObj1RcdedFlg/1 -> Compare To Zero1/1
  Constant1/1 -> Switch2/1
  Compare To Zero/1 -> Switch4/2
  Switch4/1 -> LM_OTLBufEgo1DyVarHist/1  "LM_OTLBufEgo1DyVarHist"
  Switch1/1 -> Switch4/3
  LM_OTLCurLeLaObj1Index/1 -> Compare To Zero/1
  Compare To Zero1/1 -> Switch1/2
  LM_OTLCurEgoLaObj1DyVar/1 -> Switch1/1
  Constant/1 -> Switch4/1

== system LM_LIB/LM_OTLBuf1InfoNew/LM_OTL_BufLe1StoreInfoCalc/LM_OTL_ObjSICNoCurObjInBufLe1/LM_OTL_BufL1EPInfo ==
  LM_OTLBufL1SPPos : Inport
  Signal Conversion : SignalConversion  OverrideOpt=off
  LM_OTLBufL1EPPos : Outport
  wires:
  Signal Conversion/1 -> LM_OTLBufL1EPPos/1  "LM_OTLBufL1EPPos"
  LM_OTLBufL1SPPos/1 -> Signal Conversion/1

== system LM_LIB/LM_OTLBuf1InfoNew/LM_OTL_BufLe1StoreInfoCalc/LM_OTL_ObjSICNoCurObjInBufLe1/LM_OTL_BufL1IDInfo ==
  LM_OTLCurLeLaObj1Index : Inport
  LM_OTLCurLeLaObj2Index : Inport  Port=2
  LM_OTLCurLeLaObj1RcdedFlg : Inport  Port=3
  LM_OTLCurLeLaObj1ID : Inport  Port=4
  LM_OTLCurLeLaObj2ID : Inport  Port=5
  Compare To Zero : simulink/Logic and Bit Operations/Compare To Zero  relop===  OutDataTypeStr=boolean
  Compare To Zero1 : simulink/Logic and Bit Operations/Compare To Zero  relop===  OutDataTypeStr=boolean
  Compare To Zero2 : simulink/Logic and Bit Operations/Compare To Zero  relop===  OutDataTypeStr=boolean
  Compare To Zero3 : simulink/Logic and Bit Operations/Compare To Zero  relop=~=  OutDataTypeStr=boolean
  Constant : Constant  Value=0  OutDataTypeStr=single
  Constant1 : Constant  Value=0  OutDataTypeStr=single
  Switch1 : Switch  Criteria=u2 ~= 0
  Switch2 : Switch  Criteria=u2 ~= 0
  Switch4 : Switch  Criteria=u2 ~= 0
  LM_OTLBufL1UpdateFlg : Outport
  LM_OTLBufL1ObjID : Outport  Port=2
  wires:
  Constant/1 -> Switch4/1
  LM_OTLCurLeLaObj1ID/1 -> Switch1/1
  Compare To Zero1/1 -> Switch1/2
  LM_OTLCurLeLaObj1Index/1 -> Compare To Zero/1
  Switch1/1 -> Switch4/3
  Switch4/1 -> Compare To Zero3/1, LM_OTLBufL1ObjID/1  "LM_OTLBufL1ObjID"
  Compare To Zero/1 -> Switch4/2
  Constant1/1 -> Switch2/1
  LM_OTLCurLeLaObj1RcdedFlg/1 -> Compare To Zero1/1
  LM_OTLCurLeLaObj2Index/1 -> Compare To Zero2/1
  LM_OTLCurLeLaObj2ID/1 -> Switch2/3
  Compare To Zero2/1 -> Switch2/2
  Switch2/1 -> Switch1/3
  Compare To Zero3/1 -> LM_OTLBufL1UpdateFlg/1  "LM_OTLBufL1UpdateFlg"

== system LM_LIB/LM_OTLBuf1InfoNew/LM_OTL_BufLe1StoreInfoCalc/LM_OTL_ObjSICNoCurObjInBufLe1/LM_OTL_BufL1PNumInfo ==
  LM_OTLCurLeLaObj1Index : Inport
  LM_OTLCurLeLaObj2Index : Inport  Port=2
  LM_OTLCurLeLaObj1RcdedFlg : Inport  Port=3
  Compare To Zero : simulink/Logic and Bit Operations/Compare To Zero  relop===  OutDataTypeStr=boolean
  Compare To Zero1 : simulink/Logic and Bit Operations/Compare To Zero  relop===  OutDataTypeStr=boolean
  Compare To Zero2 : simulink/Logic and Bit Operations/Compare To Zero  relop===  OutDataTypeStr=boolean
  Constant : Constant  Value=0  OutDataTypeStr=uint8
  Constant1 : Constant  Value=0  OutDataTypeStr=uint8
  Constant2 : Constant  OutDataTypeStr=uint8
  Constant3 : Constant  OutDataTypeStr=uint8
  Switch1 : Switch  Criteria=u2 ~= 0
  Switch2 : Switch  Criteria=u2 ~= 0
  Switch4 : Switch  Criteria=u2 ~= 0
  LM_OTLBufL1TPNum : Outport
  wires:
  Switch2/1 -> Switch1/3
  Switch4/1 -> LM_OTLBufL1TPNum/1  "LM_OTLBufL1TPNum"
  Compare To Zero2/1 -> Switch2/2
  Switch1/1 -> Switch4/3
  LM_OTLCurLeLaObj1RcdedFlg/1 -> Compare To Zero1/1
  LM_OTLCurLeLaObj2Index/1 -> Compare To Zero2/1
  LM_OTLCurLeLaObj1Index/1 -> Compare To Zero/1
  Constant1/1 -> Switch2/1
  Compare To Zero1/1 -> Switch1/2
  Constant/1 -> Switch4/1
  Compare To Zero/1 -> Switch4/2
  Constant2/1 -> Switch1/1
  Constant3/1 -> Switch2/3

== system LM_LIB/LM_OTLBuf1InfoNew/LM_OTL_BufLe1StoreInfoCalc/LM_OTL_ObjSICNoCurObjInBufLe1/LM_OTL_BufL1SPInfo ==
  LM_OTLCurLeLaObj1Index : Inport
  LM_OTLCurLeLaObj2Index : Inport  Port=2
  LM_OTLCurLeLaObj1RcdedFlg : Inport  Port=3
  LM_OTLBufL1LastTPValid : Inport  Port=4
  LM_OTLBufL1LastEPPos : Inport  Port=5
  Add : Sum
  Compare To Zero{,1..3} (4 alike) : simulink/Logic and Bit Operations/Compare To Zero  relop===  OutDataTypeStr=boolean
  Constant : Constant  Value=0  OutDataTypeStr=uint8
  Constant1 : Constant  Value=0  OutDataTypeStr=uint8
  Constant2 : Constant  OutDataTypeStr=uint8
  Constant3 : Constant  OutDataTypeStr=uint8
  Constant4 : Constant  Value=P_LM_OTLTPNum  OutDataTypeStr=uint8
  Relational Operator2 : RelationalOperator  Operator=>  OutDataTypeStr=boolean  RndMeth=Simplest
  Switch{,1..4} (5 alike) : Switch  Criteria=u2 ~= 0
  LM_OTLBufL1SPPos : Outport
  wires:
  Constant/1 -> Switch4/1
  Compare To Zero/1 -> Switch4/2
  Constant1/1 -> Switch2/1
  Compare To Zero1/1 -> Switch1/2
  LM_OTLCurLeLaObj2Index/1 -> Compare To Zero2/1
  Switch1/1 -> Switch4/3
  LM_OTLCurLeLaObj1RcdedFlg/1 -> Compare To Zero1/1
  LM_OTLCurLeLaObj1Index/1 -> Compare To Zero/1
  Compare To Zero2/1 -> Switch2/2
  Switch3/1 -> LM_OTLBufL1SPPos/1  "LM_OTLBufL1SPPos"
  Switch/1 -> Switch1/1
  Switch2/1 -> Switch1/3
  Add/1 -> Switch2/3, Switch/3
  LM_OTLBufL1LastTPValid/1 -> Compare To Zero3/1
  Compare To Zero3/1 -> Switch/2
  Constant2/1 -> Add/2, Switch/1
  LM_OTLBufL1LastEPPos/1 -> Add/1
  Relational Operator2/1 -> Switch3/2
  Constant3/1 -> Switch3/1
  Switch4/1 -> Switch3/3, Relational Operator2/1
  Constant4/1 -> Relational Operator2/2

== system LM_LIB/LM_OTLBuf2InfoNew/LM_OTL_BufLe1StoreInfoCalc/LM_OTL_ObjSICCurLeObj1InBufLe1/LM_OTL_BufL1DxInfo ==
  LM_OTLCurLeLaObj1Dx : Inport
  LM_OTLCurLeLaObj1RcdFlg : Inport  Port=2
  Constant : Constant  Value=0  OutDataTypeStr=single
  Switch4 : Switch  Criteria=u2 ~= 0
  LM_OTLBufL1Objdx : Outport
  wires:
  LM_OTLCurLeLaObj1Dx/1 -> Switch4/1
  LM_OTLCurLeLaObj1RcdFlg/1 -> Switch4/2
  Switch4/1 -> LM_OTLBufL1Objdx/1  "LM_OTLBufL1Objdx"
  Constant/1 -> Switch4/3

== system LM_LIB/LM_OTLBuf2InfoNew/LM_OTL_BufLe1StoreInfoCalc/LM_OTL_ObjSICCurLeObj1InBufLe1/LM_OTL_BufL1DyInfo ==
  LM_OTLCurLeLaObj1Dy : Inport
  LM_OTLCurLeLaObj1RcdFlg : Inport  Port=2
  LM_OTLCurLeLaObj1Dx : Inport  Port=3
  LM_OTLCurEgoLaObj1DyVar : Inport  Port=4
  LM_OTLCurEgoLaObj1Vy : Inport  Port=5
  LM_OTLCurEgoLaObj1VyVar : Inport  Port=6
  LM_OTLBufEgo1DyFiltHistK : Inport  Port=7
  LM_OTLBufEgo1DyVarHistK : Inport  Port=8
  psiDt : Inport  Port=9
  tDt : Inport  Port=10
  Constant : Constant  Value=0  OutDataTypeStr=single
  Constant1 : Constant  Value=0.5  OutDataTypeStr=single
  MATLAB Function : MATLAB Function  TreatAsAtomicUnit=on
  Switch1 : Switch  Criteria=u2 ~= 0
  Switch4 : Switch  Criteria=u2 ~= 0
  LM_OTLBufL1ObjDy : Outport
  LM_OTLBufEgo1DyVarHist : Outport  Port=2
  wires:
  Constant/1 -> Switch4/3
  Switch4/1 -> LM_OTLBufL1ObjDy/1  "LM_OTLBufL1ObjDy"
  LM_OTLCurLeLaObj1Dy/1 -> MATLAB Function/2(dy)
  LM_OTLCurLeLaObj1RcdFlg/1 -> Switch1/2, Switch4/2
  LM_OTLCurEgoLaObj1DyVar/1 -> MATLAB Function/3(varDy)
  LM_OTLCurEgoLaObj1Vy/1 -> MATLAB Function/4(vy)
  LM_OTLCurEgoLaObj1VyVar/1 -> MATLAB Function/5(varVy)
  LM_OTLCurLeLaObj1Dx/1 -> MATLAB Function/1(dx)
  LM_OTLBufEgo1DyFiltHistK/1 -> MATLAB Function/8(dyHist)
  Constant1/1 -> Switch1/3, MATLAB Function/9(varDyHist)
  Switch1/1 -> LM_OTLBufEgo1DyVarHist/1  "LM_OTLBufL1ObjDy"
  MATLAB Function/2(varDyFilt) -> Switch1/1
  MATLAB Function/1(dyFilt) -> Switch4/1
  psiDt/1 -> MATLAB Function/6(psiDt)
  tDt/1 -> MATLAB Function/7(tDt)

== system LM_LIB/LM_OTLBuf2InfoNew/LM_OTL_BufLe1StoreInfoCalc/LM_OTL_ObjSICCurLeObj1InBufLe1/LM_OTL_BufL1EPInfo ==
  note: P_LM_OTLTPNum
  LM_OTLCurLeLaObj1RcdFlg : Inport
  LM_OTLBufL1EPPosK1 : Inport  Port=2
  Add : Sum
  Constant : Constant  OutDataTypeStr=uint8
  Constant1 : Constant  Value=P_LM_OTLTPNum  OutDataTypeStr=uint8
  Constant2 : Constant  OutDataTypeStr=uint8
  Relational Operator : RelationalOperator  Operator=>  OutDataTypeStr=boolean  RndMeth=Simplest
  Switch1 : Switch  Criteria=u2 ~= 0
  Switch4 : Switch  Criteria=u2 ~= 0
  LM_OTLBufL1EPPos : Outport
  wires:
  Constant/1 -> Add/2
  LM_OTLCurLeLaObj1RcdFlg/1 -> Switch4/2
  LM_OTLBufL1EPPosK1/1 -> Switch4/3, Add/1
  Switch1/1 -> LM_OTLBufL1EPPos/1  "LM_OTLBufL1EPPos"
  Relational Operator/1 -> Switch1/2
  Switch4/1 -> Switch1/3, Relational Operator/1
  Constant1/1 -> Relational Operator/2
  Constant2/1 -> Switch1/1
  Add/1 -> Switch4/1

== system LM_LIB/LM_OTLBuf2InfoNew/LM_OTL_BufLe1StoreInfoCalc/LM_OTL_ObjSICCurLeObj1InBufLe1/LM_OTL_BufL1IDInfo ==
  LM_OTLCurLeLaObj1ID : Inport
  Signal Conversion : SignalConversion  OverrideOpt=off
  LM_OTLBufL1ObjID : Outport
  wires:
  LM_OTLCurLeLaObj1ID/1 -> Signal Conversion/1
  Signal Conversion/1 -> LM_OTLBufL1ObjID/1  "LM_OTLBufL1ObjID"

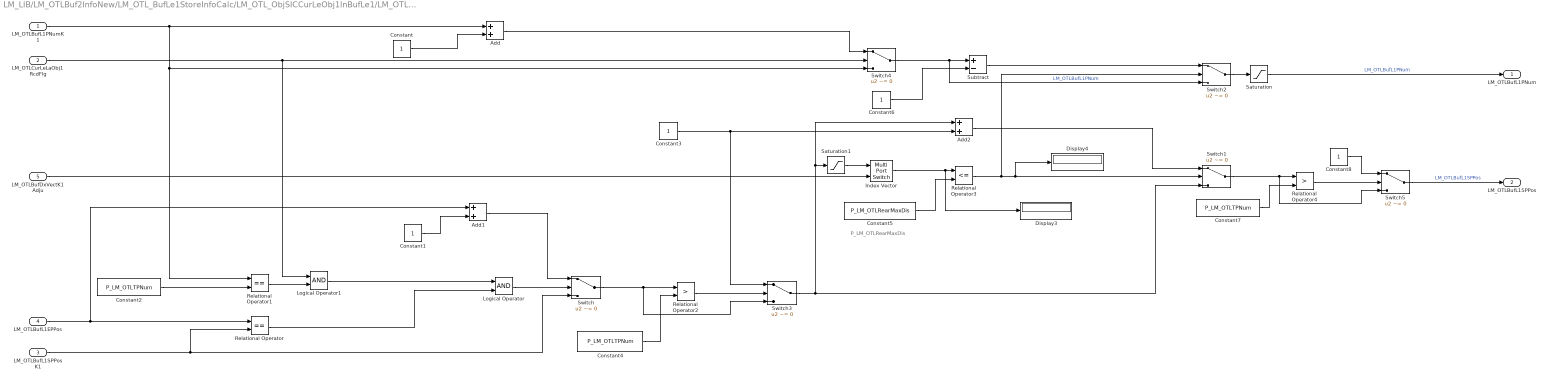
== system LM_LIB/LM_OTLBuf2InfoNew/LM_OTL_BufLe1StoreInfoCalc/LM_OTL_ObjSICCurLeObj1InBufLe1/LM_OTL_BufL1PNumAndSPInfo ==
  note: P_LM_OTLRearMaxDis
  LM_OTLBufL1PNumK1 : Inport
  LM_OTLCurLeLaObj1RcdFlg : Inport  Port=2
  LM_OTLBufL1SPPosK1 : Inport  Port=3
  LM_OTLBufL1EPPos : Inport  Port=4
  LM_OTLBufDxVectK1Adju : Inport  Port=5
  Add : Sum
  Add1 : Sum
  Add2 : Sum
  Constant{,1,3,6,8} (5 alike) : Constant  OutDataTypeStr=uint8
  Constant2 : Constant  Value=P_LM_OTLTPNum  OutDataTypeStr=uint8
  Constant4 : Constant  Value=P_LM_OTLTPNum  OutDataTypeStr=uint8
  Constant5 : Constant  Value=P_LM_OTLRearMaxDis
  Constant7 : Constant  Value=P_LM_OTLTPNum  OutDataTypeStr=uint8
  Display3 : Display
  Display4 : Display
  Index Vector : MultiPortSwitch  Inputs=1
  Logical Operator : Logic  AllPortsSameDT=off  OutDataTypeStr=boolean
  Logical Operator1 : Logic  AllPortsSameDT=off  OutDataTypeStr=boolean
  Relational Operator : RelationalOperator  Operator===  OutDataTypeStr=boolean  RndMeth=Simplest
  Relational Operator1 : RelationalOperator  Operator===  OutDataTypeStr=boolean  RndMeth=Simplest
  Relational Operator2 : RelationalOperator  Operator=>  OutDataTypeStr=boolean  RndMeth=Simplest
  Relational Operator3 : RelationalOperator  Operator=<=  OutDataTypeStr=boolean  RndMeth=Simplest
  Relational Operator4 : RelationalOperator  Operator=>  OutDataTypeStr=boolean  RndMeth=Simplest
  Saturation : Saturate  UpperLimit=80  LowerLimit=0
  Saturation1 : Saturate  UpperLimit=80  LowerLimit=0
  Subtract : Sum  Inputs=+-
  Switch{,1..5} (6 alike) : Switch  Criteria=u2 ~= 0
  LM_OTLBufL1PNum : Outport
  LM_OTLBufL1SPPos : Outport  Port=2
  wires:
  Saturation/1 -> LM_OTLBufL1PNum/1  "LM_OTLBufL1PNum"
  LM_OTLCurLeLaObj1RcdFlg/1 -> Logical Operator1/1, Switch4/2
  Switch2/1 -> Saturation/1
  Constant/1 -> Add/2
  Add/1 -> Switch4/1
  Constant2/1 -> Relational Operator1/2
  Constant3/1 -> Switch3/1, Add2/2
  Constant4/1 -> Relational Operator2/2
  Add1/1 -> Switch/1
  Switch/1 -> Switch3/3, Relational Operator2/1
  Relational Operator2/1 -> Switch3/2
  LM_OTLBufL1SPPosK1/1 -> Switch/3, Relational Operator/2
  Relational Operator1/1 -> Logical Operator1/2
  Logical Operator/1 -> Switch/2
  LM_OTLBufL1EPPos/1 -> Relational Operator/1, Add1/1
  Relational Operator/1 -> Logical Operator/2
  LM_OTLBufL1PNumK1/1 -> Add/1, Relational Operator1/1, Switch4/3
  Switch3/1 -> Switch1/3, Add2/1, Saturation1/1
  Constant1/1 -> Add1/2
  LM_OTLBufDxVectK1Adju/1 -> Index Vector/2
  Index Vector/1 -> Display3/1, Relational Operator3/1
  Constant5/1 -> Relational Operator3/2
  Relational Operator3/1 -> Switch2/2, Display4/1, Switch1/2
  Switch5/1 -> LM_OTLBufL1SPPos/1  "LM_OTLBufL1SPPos"
  Add2/1 -> Switch1/1
  Subtract/1 -> Switch2/1
  Saturation1/1 -> Index Vector/1
  Logical Operator1/1 -> Logical Operator/1
  Switch4/1 -> Switch2/3, Subtract/1  "LM_OTLBufL1PNum"
  Constant6/1 -> Subtract/2
  Switch1/1 -> Switch5/3, Relational Operator4/1
  Relational Operator4/1 -> Switch5/2
  Constant7/1 -> Relational Operator4/2
  Constant8/1 -> Switch5/1

== system LM_LIB/LM_OTLBuf2InfoNew/LM_OTL_BufLe1StoreInfoCalc/LM_OTL_ObjSICCurLeObj1InBufLe1/LM_OTL_BufL1UpdateFlg ==
  LM_OTLCurLeLaObj1RcdFlg : Inport
  Signal Conversion : SignalConversion  OverrideOpt=off
  LM_OTLBufL1UpdateFlg : Outport
  wires:
  LM_OTLCurLeLaObj1RcdFlg/1 -> Signal Conversion/1
  Signal Conversion/1 -> LM_OTLBufL1UpdateFlg/1  "LM_OTLBufL1UpdateFlg"

== system LM_LIB/LM_OTLBuf2InfoNew/LM_OTL_BufLe1StoreInfoCalc/LM_OTL_ObjSICCurLeObj2InBufLe1/LM_OTL_BufL1DxInfo ==
  LM_OTLCurLeLaObj1Dx : Inport
  LM_OTLCurLeLaObj1RcdFlg : Inport  Port=2
  Constant : Constant  Value=0  OutDataTypeStr=single
  Switch4 : Switch  Criteria=u2 ~= 0
  LM_OTLBufL1Objdx : Outport
  wires:
  LM_OTLCurLeLaObj1Dx/1 -> Switch4/1
  LM_OTLCurLeLaObj1RcdFlg/1 -> Switch4/2
  Switch4/1 -> LM_OTLBufL1Objdx/1  "LM_OTLBufL1Objdx"
  Constant/1 -> Switch4/3

== system LM_LIB/LM_OTLBuf2InfoNew/LM_OTL_BufLe1StoreInfoCalc/LM_OTL_ObjSICCurLeObj2InBufLe1/LM_OTL_BufL1DyInfo ==
  LM_OTLCurEgoLaObj2Dx : Inport
  LM_OTLCurLeLaObj1Dy : Inport  Port=2
  LM_OTLCurLeLaObj1RcdFlg : Inport  Port=3
  LM_OTLCurEgoLaObj2DyVar : Inport  Port=4
  LM_OTLCurEgoLaObj2Vy : Inport  Port=5
  LM_OTLCurEgoLaObj2VyVar : Inport  Port=6
  LM_OTLBufEgo1DyFiltHistK : Inport  Port=7
  LM_OTLBufEgo1DyVarHistK : Inport  Port=8
  psiDt : Inport  Port=9
  tDt : Inport  Port=10
  Constant : Constant  Value=0  OutDataTypeStr=single
  Constant1 : Constant  Value=0.5  OutDataTypeStr=single
  MATLAB Function : MATLAB Function  TreatAsAtomicUnit=on
  Switch1 : Switch  Criteria=u2 ~= 0
  Switch4 : Switch  Criteria=u2 ~= 0
  LM_OTLBufL1ObjDy : Outport
  LM_OTLBufEgo1DyVarHist : Outport  Port=2
  wires:
  Constant/1 -> Switch4/3
  Switch4/1 -> LM_OTLBufL1ObjDy/1  "LM_OTLBufL1ObjDy"
  LM_OTLCurLeLaObj1Dy/1 -> MATLAB Function/2(dy)
  LM_OTLCurLeLaObj1RcdFlg/1 -> Switch1/2, Switch4/2
  LM_OTLCurEgoLaObj2VyVar/1 -> MATLAB Function/5(varVy)
  LM_OTLCurEgoLaObj2Vy/1 -> MATLAB Function/4(vy)
  LM_OTLCurEgoLaObj2DyVar/1 -> MATLAB Function/3(varDy)
  LM_OTLCurEgoLaObj2Dx/1 -> MATLAB Function/1(dx)
  MATLAB Function/1(dyFilt) -> Switch4/1
  MATLAB Function/2(varDyFilt) -> Switch1/1
  Constant1/1 -> MATLAB Function/9(varDyHist), Switch1/3
  psiDt/1 -> MATLAB Function/6(psiDt)
  tDt/1 -> MATLAB Function/7(tDt)
  LM_OTLBufEgo1DyFiltHistK/1 -> MATLAB Function/8(dyHist)
  Switch1/1 -> LM_OTLBufEgo1DyVarHist/1  "LM_OTLBufEgo1DyVarHist"

== system LM_LIB/LM_OTLBuf2InfoNew/LM_OTL_BufLe1StoreInfoCalc/LM_OTL_ObjSICCurLeObj2InBufLe1/LM_OTL_BufL1EPInfo ==
  note: P_LM_OTLTPNum
  LM_OTLCurLeLaObj1RcdFlg : Inport
  LM_OTLBufL1EPPosK1 : Inport  Port=2
  Add : Sum
  Constant : Constant  OutDataTypeStr=uint8
  Constant1 : Constant  Value=80  OutDataTypeStr=uint8
  Constant2 : Constant  OutDataTypeStr=uint8
  Relational Operator : RelationalOperator  Operator=>  OutDataTypeStr=boolean  RndMeth=Simplest
  Switch1 : Switch  Criteria=u2 ~= 0
  Switch4 : Switch  Criteria=u2 ~= 0
  LM_OTLBufL1EPPos : Outport
  wires:
  Constant/1 -> Add/2
  LM_OTLCurLeLaObj1RcdFlg/1 -> Switch4/2
  LM_OTLBufL1EPPosK1/1 -> Switch4/3, Add/1
  Switch1/1 -> LM_OTLBufL1EPPos/1  "LM_OTLBufL1EPPos"
  Relational Operator/1 -> Switch1/2
  Switch4/1 -> Switch1/3, Relational Operator/1
  Constant1/1 -> Relational Operator/2
  Constant2/1 -> Switch1/1
  Add/1 -> Switch4/1

== system LM_LIB/LM_OTLBuf2InfoNew/LM_OTL_BufLe1StoreInfoCalc/LM_OTL_ObjSICCurLeObj2InBufLe1/LM_OTL_BufL1IDInfo ==
  LM_OTLCurLeLaObj1ID : Inport
  Signal Conversion : SignalConversion  OverrideOpt=off
  LM_OTLBufL1ObjID : Outport
  wires:
  LM_OTLCurLeLaObj1ID/1 -> Signal Conversion/1
  Signal Conversion/1 -> LM_OTLBufL1ObjID/1  "LM_OTLBufL1ObjID"

== system LM_LIB/LM_OTLBuf2InfoNew/LM_OTL_BufLe1StoreInfoCalc/LM_OTL_ObjSICCurLeObj2InBufLe1/LM_OTL_BufL1PNumAndSPInfo ==
  note: P_LM_OTLRearMaxDis
  LM_OTLBufL1PNumK1 : Inport
  LM_OTLCurLeLaObj2RcdFlg : Inport  Port=2
  LM_OTLBufL1SPPosK1 : Inport  Port=3
  LM_OTLBufL1EPPos : Inport  Port=4
  LM_OTLBufDxVectK1Adju : Inport  Port=5
  Add : Sum
  Add1 : Sum
  Add2 : Sum
  Constant{,1,3,7} (4 alike) : Constant  OutDataTypeStr=uint8
  Constant2 : Constant  Value=P_LM_OTLTPNum  OutDataTypeStr=uint8
  Constant4 : Constant  Value=P_LM_OTLTPNum  OutDataTypeStr=uint8
  Constant5 : Constant  Value=P_LM_OTLRearMaxDis
  Constant6 : Constant  Value=P_LM_OTLTPNum  OutDataTypeStr=uint8
  Index Vector : MultiPortSwitch  Inputs=1
  Logical Operator : Logic  AllPortsSameDT=off  OutDataTypeStr=boolean
  Logical Operator1 : Logic  AllPortsSameDT=off  OutDataTypeStr=boolean
  Relational Operator : RelationalOperator  Operator===  OutDataTypeStr=boolean  RndMeth=Simplest
  Relational Operator1 : RelationalOperator  Operator===  OutDataTypeStr=boolean  RndMeth=Simplest
  Relational Operator2 : RelationalOperator  Operator=>  OutDataTypeStr=boolean  RndMeth=Simplest
  Relational Operator3 : RelationalOperator  Operator=<=  OutDataTypeStr=boolean  RndMeth=Simplest
  Relational Operator4 : RelationalOperator  Operator=>  OutDataTypeStr=boolean  RndMeth=Simplest
  Saturation : Saturate  UpperLimit=80  LowerLimit=0
  Saturation1 : Saturate  UpperLimit=80  LowerLimit=1
  Subtract : Sum  Inputs=+-
  Switch{,1..5} (6 alike) : Switch  Criteria=u2 ~= 0
  LM_OTLBufL1PNum : Outport
  LM_OTLBufL1SPPos : Outport  Port=2
  wires:
  Switch5/1 -> LM_OTLBufL1SPPos/1  "LM_OTLBufL1SPPos"
  LM_OTLBufL1PNumK1/1 -> Add/1, Switch4/3, Relational Operator1/1
  LM_OTLBufL1SPPosK1/1 -> Switch/3, Relational Operator/2
  Relational Operator2/1 -> Switch3/2
  Switch/1 -> Switch3/3, Relational Operator2/1
  Constant3/1 -> Add2/2, Switch3/1
  Relational Operator/1 -> Logical Operator/2
  Add1/1 -> Switch/1
  Relational Operator1/1 -> Logical Operator1/2
  Relational Operator3/1 -> Switch2/2, Switch1/2
  Add2/1 -> Switch1/1
  Index Vector/1 -> Relational Operator3/1
  LM_OTLBufL1EPPos/1 -> Relational Operator/1, Add1/1
  Constant1/1 -> Add1/2
  Constant/1 -> Subtract/2, Add/2
  LM_OTLCurLeLaObj2RcdFlg/1 -> Logical Operator1/1, Switch4/2
  Saturation/1 -> LM_OTLBufL1PNum/1  "LM_OTLBufL1PNum"
  Constant4/1 -> Relational Operator2/2
  Constant5/1 -> Relational Operator3/2
  Switch3/1 -> Switch1/3, Add2/1, Saturation1/1
  LM_OTLBufDxVectK1Adju/1 -> Index Vector/2
  Logical Operator/1 -> Switch/2
  Subtract/1 -> Switch2/1
  Saturation1/1 -> Index Vector/1
  Constant2/1 -> Relational Operator1/2
  Logical Operator1/1 -> Logical Operator/1
  Add/1 -> Switch4/1
  Switch2/1 -> Saturation/1  "LM_OTLBufL1PNum"
  Switch4/1 -> Subtract/1, Switch2/3  "LM_OTLBufL1PNum"
  Switch1/1 -> Switch5/3, Relational Operator4/1
  Relational Operator4/1 -> Switch5/2
  Constant6/1 -> Relational Operator4/2
  Constant7/1 -> Switch5/1

== system LM_LIB/LM_OTLBuf2InfoNew/LM_OTL_BufLe1StoreInfoCalc/LM_OTL_ObjSICCurLeObj2InBufLe1/LM_OTL_BufL1UpdateFlg ==
  LM_OTLCurLeLaObj1RcdFlg : Inport
  Signal Conversion : SignalConversion  OverrideOpt=off
  LM_OTLBufL1UpdateFlg : Outport
  wires:
  LM_OTLCurLeLaObj1RcdFlg/1 -> Signal Conversion/1
  Signal Conversion/1 -> LM_OTLBufL1UpdateFlg/1  "LM_OTLBufL1UpdateFlg"

== system LM_LIB/LM_OTLBuf2InfoNew/LM_OTL_BufLe1StoreInfoCalc/LM_OTL_ObjSICNoCurObjInBufLe1/LM_OTL_BufL1IDInfo1 ==
  LM_OTLBuf1ID : Inport
  LM_OTLCurLeLaObj1Index : Inport  Port=2
  LM_OTLCurLeLaObj2Index : Inport  Port=3
  LM_OTLCurLeLaObj1RcdedFlg : Inport  Port=4
  LM_OTLCurLeLaObj1ID : Inport  Port=5
  LM_OTLCurLeLaObj2ID : Inport  Port=6
  Compare To Zero : simulink/Logic and Bit Operations/Compare To Zero  relop===  OutDataTypeStr=boolean
  Compare To Zero1 : simulink/Logic and Bit Operations/Compare To Zero  relop===  OutDataTypeStr=boolean
  Compare To Zero2 : simulink/Logic and Bit Operations/Compare To Zero  relop===  OutDataTypeStr=boolean
  Compare To Zero3 : simulink/Logic and Bit Operations/Compare To Zero  relop=~=  OutDataTypeStr=boolean
  Constant : Constant  Value=0  OutDataTypeStr=single
  Constant1 : Constant  Value=0  OutDataTypeStr=single
  Relational Operator1 : RelationalOperator  Operator===  OutDataTypeStr=boolean  RndMeth=Simplest
  Switch{1..2,4..5} (4 alike) : Switch  Criteria=u2 ~= 0
  LM_OTLBuf2UpdateFlg : Outport
  LM_OTLBuf2ObjID : Outport  Port=2
  wires:
  Switch5/1 -> Switch4/3  "LM_OTLBufL1ObjID"
  Relational Operator1/1 -> Switch5/2
  Switch1/1 -> Relational Operator1/2, Switch5/3
  LM_OTLBuf1ID/1 -> Relational Operator1/1
  Switch2/1 -> Switch1/3, Switch5/1
  Compare To Zero3/1 -> LM_OTLBuf2UpdateFlg/1
  Compare To Zero2/1 -> Switch2/2
  LM_OTLCurLeLaObj2ID/1 -> Switch2/3
  LM_OTLCurLeLaObj2Index/1 -> Compare To Zero2/1
  LM_OTLCurLeLaObj1RcdedFlg/1 -> Compare To Zero1/1
  Constant1/1 -> Switch2/1
  Compare To Zero/1 -> Switch4/2
  Switch4/1 -> Compare To Zero3/1, LM_OTLBuf2ObjID/1  "LM_OTLBuf1ObjID"
  LM_OTLCurLeLaObj1Index/1 -> Compare To Zero/1
  Compare To Zero1/1 -> Switch1/2
  LM_OTLCurLeLaObj1ID/1 -> Switch1/1
  Constant/1 -> Switch4/1

== system LM_LIB/LM_OTLBuf2InfoNew/LM_OTL_BufLe1StoreInfoCalc/LM_OTL_ObjSICNoCurObjInBufLe1/LM_OTL_BufL1PNumInfo1 ==
  LM_OTLBufL2ObjID : Inport
  Compare To Zero : simulink/Logic and Bit Operations/Compare To Zero  relop===  OutDataTypeStr=boolean
  Constant : Constant  Value=0  OutDataTypeStr=uint8
  Constant2 : Constant  OutDataTypeStr=uint8
  Switch4 : Switch  Criteria=u2 ~= 0
  LM_OTLBuf2TPNum : Outport
  wires:
  Compare To Zero/1 -> Switch4/2
  Constant/1 -> Switch4/1
  LM_OTLBufL2ObjID/1 -> Compare To Zero/1
  Constant2/1 -> Switch4/3
  Switch4/1 -> LM_OTLBuf2TPNum/1  "LM_OTLBuf2TPNum"

== system LM_LIB/LM_OTLBuf2InfoNew/LM_OTL_BufLe1StoreInfoCalc/LM_OTL_ObjSICNoCurObjInBufLe1/LM_OTL_BufL1SPInfo1 ==
  LM_OTLBufL2ObjID : Inport
  LM_OTLBufL2LastTPValid : Inport  Port=2
  LM_OTLBufL2LastEPPos : Inport  Port=3
  Add : Sum
  Compare To Zero : simulink/Logic and Bit Operations/Compare To Zero  relop===  OutDataTypeStr=boolean
  Compare To Zero3 : simulink/Logic and Bit Operations/Compare To Zero  relop===  OutDataTypeStr=boolean
  Constant : Constant  Value=0  OutDataTypeStr=uint8
  Constant1 : Constant  OutDataTypeStr=uint8
  Constant2 : Constant  OutDataTypeStr=uint8
  Constant3 : Constant  Value=P_LM_OTLTPNum  OutDataTypeStr=uint8
  Relational Operator2 : RelationalOperator  Operator=>  OutDataTypeStr=boolean  RndMeth=Simplest
  Switch : Switch  Criteria=u2 ~= 0
  Switch1 : Switch  Criteria=u2 ~= 0
  Switch4 : Switch  Criteria=u2 ~= 0
  LM_OTLBuf2SPPos : Outport
  wires:
  Relational Operator2/1 -> Switch1/2
  Switch4/1 -> Relational Operator2/1, Switch1/3
  Constant3/1 -> Relational Operator2/2
  Constant1/1 -> Switch1/1
  LM_OTLBufL2LastEPPos/1 -> Add/1
  Constant2/1 -> Switch/1, Add/2
  Compare To Zero3/1 -> Switch/2
  LM_OTLBufL2LastTPValid/1 -> Compare To Zero3/1
  Add/1 -> Switch/3
  Switch1/1 -> LM_OTLBuf2SPPos/1  "LM_OTLBuf2SPPos"
  LM_OTLBufL2ObjID/1 -> Compare To Zero/1
  Switch/1 -> Switch4/3
  Compare To Zero/1 -> Switch4/2
  Constant/1 -> Switch4/1

== system LM_LIB/LM_OTLBuf2InfoNew/LM_OTL_BufLe1StoreInfoCalc/LM_OTL_ObjSICNoCurObjInBufLe1/LM_OTL_BufL2EPInfo ==
  LM_OTLBufL2SPPos : Inport
  Signal Conversion : SignalConversion  OverrideOpt=off
  LM_OTLBuf2EPPos : Outport
  wires:
  LM_OTLBufL2SPPos/1 -> Signal Conversion/1
  Signal Conversion/1 -> LM_OTLBuf2EPPos/1  "LM_OTLBuf2EPPos"

== system LM_LIB/LM_OTLBuf2InfoNew/LM_OTL_BufLe1StoreInfoCalc/LM_OTL_ObjSICNoCurObjInBufLe1/LM_OTL_BufL2PosInfo ==
  LM_OTLBufL2ObjID : Inport
  LM_OTLCurLeLaObj1ID : Inport  Port=2
  LM_OTLCurLeLaObj2ID : Inport  Port=3
  LM_OTLCurLeLaObj1Dx : Inport  Port=4
  LM_OTLCurLeLaObj2Dx : Inport  Port=5
  LM_OTLCurLeLaObj1Dy : Inport  Port=6
  LM_OTLCurLeLaObj2Dy : Inport  Port=7
  LM_OTLCurEgoLaObj1DyVar : Inport  Port=8
  LM_OTLCurEgoLaObj2DyVar : Inport  Port=9
  Compare To Zero : simulink/Logic and Bit Operations/Compare To Zero  relop===  OutDataTypeStr=boolean
  Constant{,1..3} (4 alike) : Constant  Value=0  OutDataTypeStr=single
  DocBlock : simulink/Model-Wide Utilities/DocBlock  DocumentType=Text
      content=|
      | 1. 功能描述
      |    该模块主要功能
      | 2. 算法说明
      | 2.1 当左车道最近目标索引为0时，即左车道无目标，输出0
      | 2.2 当左车道最近目标索引不为0时
      |     2.2.1 如果左车道最近目标ID未在buffer中存储，则输出左车道最近目标的dx
      |     2.2.2 如果左车道最近目标ID已经在buffer中存储
      |           2.2.2.1 如果左车道第二近目标ID不为0，则输出左车道第二近目标dx
      |           2.2.2.2 如果左车道第二近目标ID为0，则输出0
  Relational Operator : RelationalOperator  Operator===  OutDataTypeStr=boolean  RndMeth=Simplest
  Relational Operator1 : RelationalOperator  Operator===  OutDataTypeStr=boolean  RndMeth=Simplest
  Switch{1..9} (9 alike) : Switch  Criteria=u2 ~= 0
  LM_OTLBuf2Objdx : Outport
  LM_OTLBuf2Objdy : Outport  Port=2
  LM_OTLBuf2DyVarHist : Outport  Port=3
  wires:
  Switch5/1 -> LM_OTLBuf2Objdy/1  "LM_OTLBuf2Objdy"
  Constant2/1 -> Switch6/3
  Switch6/1 -> Switch3/3
  LM_OTLCurLeLaObj2Dy/1 -> Switch6/1
  Switch3/1 -> Switch5/3
  LM_OTLCurLeLaObj1Dy/1 -> Switch3/1
  Constant1/1 -> Switch2/3
  LM_OTLCurLeLaObj2ID/1 -> Relational Operator1/2
  Relational Operator/1 -> Switch1/2, Switch8/2, Switch3/2
  LM_OTLCurLeLaObj1ID/1 -> Relational Operator/2
  Switch2/1 -> Switch1/3
  LM_OTLCurLeLaObj2Dx/1 -> Switch2/1
  Relational Operator1/1 -> Switch9/2, Switch2/2, Switch6/2
  LM_OTLCurLeLaObj1Dx/1 -> Switch1/1
  Constant/1 -> Switch4/1, Switch5/1, Switch7/1
  Compare To Zero/1 -> Switch4/2, Switch5/2, Switch7/2
  LM_OTLBufL2ObjID/1 -> Compare To Zero/1, Relational Operator1/1, Relational Operator/1
  Switch4/1 -> LM_OTLBuf2Objdx/1  "LM_OTLBuf2Objdx"
  Switch1/1 -> Switch4/3
  Switch8/1 -> Switch7/3
  LM_OTLCurEgoLaObj1DyVar/1 -> Switch8/1
  Switch7/1 -> LM_OTLBuf2DyVarHist/1  "LM_OTLBuf2DyVarHist"
  Switch9/1 -> Switch8/3
  LM_OTLCurEgoLaObj2DyVar/1 -> Switch9/1
  Constant3/1 -> Switch9/3
